simulink model "Client"  (R2016a)
settings: Solver=VariableStepAuto  StartTime=0.0  StopTime=0  RelTol=1e-3
settings Model: Creator=Hilals  LastModifiedBy=Hilals

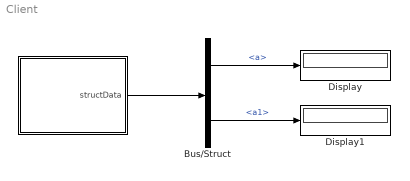
== system Client ==
  " " : MATLAB Function  TreatAsAtomicUnit=on  mask(TcpIpReceiveClient){IP=uint8('127.0.0.1'), Port=47806}
      mask prompts: IP "Remote IP Address"; Port "Remote Port"
      mask help: Receive Data from Server Side
  Bus/Struct : BusSelector  OutputSignals=a,a1
  Display : Display
  Display1 : Display
  wires:
  Bus/Struct/2 -> Display1/1  "<a1>"
  Bus/Struct/1 -> Display/1  "<a>"
  " "/1(structData) -> Bus/Struct/1

== matlab function Client/  ==
  data: IP parameter; Port parameter; structData output Bus: Bus
function structData = fcn(  IP, Port)
coder.extrinsic('tcpip'); % codegen
coder.extrinsic('fread'); % codegen
coder.extrinsic('num2cell'); % codegen
coder.extrinsic('cell2struct'); % codegen

% Char does not supported by MATLAB. Input Parameter from Simulink is uint8!!
% for this reason;
ipAddress = char(IP);

%% Tcp\Ip
t = tcpip(ipAddress,Port,'NetworkRole','client');
fopen(t);
pause(0.2); % delay


% If you send a value that is lower than 256, you could fread(t).
% or use the latest version. (2016b is possible.)
receivedData = fread(t,2,'double'); % 2 = t.BytesAvailable/8.
                                    % Because number of double variables is 2.
                                    % But t.BytesAvailable is not supported.
%% matrix --> cell array --> struct
% 2016a MATLAB problem. If you have 2016b or latest version, 
% you could use json format to receive struct data (bkz:jsonencode,jsondecode)
% [n,d] = size(receivedData);
cellData = num2cell(receivedData);
fields = {'a', 'a1'};
structData = cell2struct(cellData,fields,1);
